simulink model "QC_Test2"  (R2019a)
settings: Solver=FixedStepAuto  StartTime=0.0  StopTime=inf  RelTol=1e-3  EnableMultiTasking=on
libraries: arduinolib x8, simulink x6
settings Model: SimulationMode=external  ExtModeTrigDuration=2  Creator=chait  LastModifiedBy=DINESH
settings OptimizationCC: EnhancedBackFolding=on  PassReuseOutputArgsAs=Individual arguments  MaxStackSize=64  OptimizeBlockOrder=speed  DifferentSizesBufferReuse=on  OptimizationCustomize=off
settings DebuggingCC: ParameterTunabilityLossMsg=error
settings HardwareCC: ProdBitPerInt=16  ProdBitPerPointer=16  ProdBitPerSizeT=16  ProdBitPerPtrDiffT=16  ProdLargestAtomicFloat=None  ProdWordSize=8  ProdHWDeviceType=Atmel->AVR
settings SFSimCC: MATLABDynamicMemAlloc=off
settings RTWCC: SystemTargetFile=ert.tlc  HardwareBoard=Arduino Mega 2560  TLCOptions=-aInlineSetEventsForThisBaseRateFcn=TLC_FALSE -aSuppressMultiTaskScheduler=TLC_FALSE -aRateBasedStepFcn=1  TemplateMakefile=ert_default_tmf  GenerateReport=on  Toolchain=Arduino AVR  BuildConfiguration=Faster Runs  IncludeHyperlinkInReport=on  LaunchReport=on  GenerateTraceInfo=on  GenerateTraceReport=on  GenerateTraceReportSl=on  GenerateTraceReportSf=on  GenerateTraceReportEml=on
settings CodeAppCC: ForceParamTrailComments=on  IgnoreCustomStorageClasses=off  OperatorAnnotations=on  SimulinkDataObjDesc=on  SFDataObjDesc=on  InsertBlockDesc=on
settings ERTTargetCC: SupportContinuousTime=on  SupportVariableSizeSignals=on  ExtMode=on  ExtModeStaticAllocSize=2048  ExtModeMexArgs='127.0.0.1' 0 17725

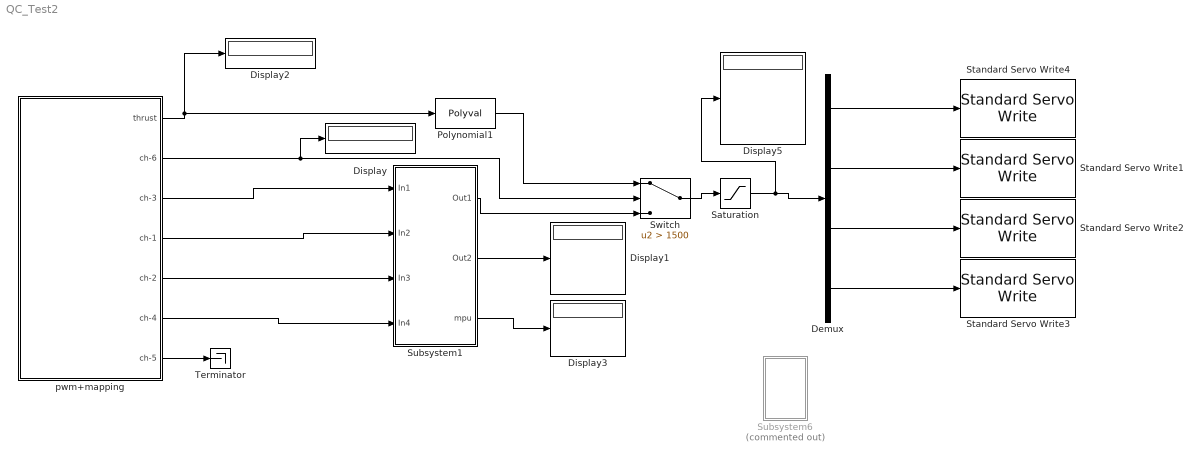
== system QC_Test2 ==
  Demux : Demux
  Display{,1..3,5} (5 alike) : Display
  Polynomial1 : Polyval  Coefs=|
      | [0.097
      |   -52]
  Saturation : Saturate  UpperLimit=142  LowerLimit=45
  Standard Servo Write1 : arduinolib/Standard Servo Write  pinNumber=6  ServoIndex=0  blockPlatform=ARDUINO
      settings: SourceProductName=Simulink Support Package for Arduino Hardware
  Standard Servo Write2 : arduinolib/Standard Servo Write  pinNumber=7  ServoIndex=1  blockPlatform=ARDUINO
      settings: SourceProductName=Simulink Support Package for Arduino Hardware
  Standard Servo Write3 : arduinolib/Standard Servo Write  pinNumber=8  ServoIndex=2  blockPlatform=ARDUINO
      settings: SourceProductName=Simulink Support Package for Arduino Hardware
  Standard Servo Write4 : arduinolib/Standard Servo Write  pinNumber=2  ServoIndex=3  blockPlatform=ARDUINO
      settings: SourceProductName=Simulink Support Package for Arduino Hardware
  Subsystem1 : Subsystem
  Subsystem6 : Subsystem  Commented=on
  Switch : Switch  Criteria=u2 > Threshold  Threshold=1500
  Terminator : Terminator
  pwm+mapping : Subsystem
  wires:
  Subsystem1/1(Out1) -> Switch/3
  Demux/3 -> Standard Servo Write2/1
  Demux/1 -> Standard Servo Write4/1
  pwm+mapping/6(ch-4) -> Subsystem1/4(In4)
  pwm+mapping/5(ch-2) -> Subsystem1/3(In3)
  Subsystem1/3(mpu) -> Display3/1
  pwm+mapping/2(ch-6) -> Display/1, Switch/2
  Polynomial1/1 -> Switch/1
  Switch/1 -> Saturation/1
  Demux/4 -> Standard Servo Write3/1
  Demux/2 -> Standard Servo Write1/1
  Saturation/1 -> Display5/1, Demux/1
  pwm+mapping/3(ch-3) -> Subsystem1/1(In1)
  pwm+mapping/1("thrust ") -> Display2/1, Polynomial1/1
  Subsystem1/2(Out2) -> Display1/1
  pwm+mapping/4(ch-1) -> Subsystem1/2(In2)
  pwm+mapping/7(ch-5) -> Terminator/1

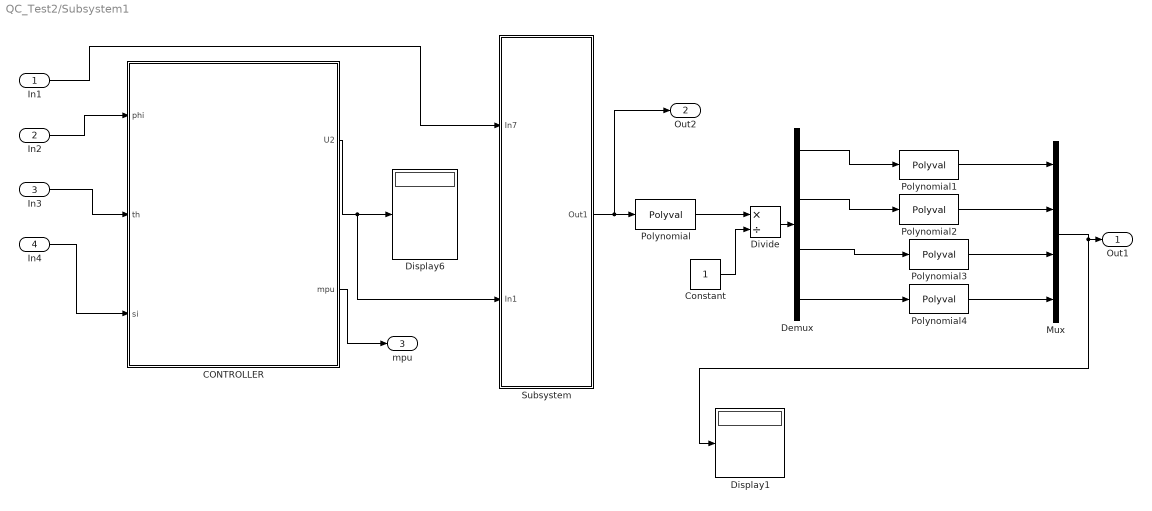
== system QC_Test2/Subsystem1 ==
  In1 : Inport
  In2 : Inport  Port=2
  In3 : Inport  Port=3
  In4 : Inport  Port=4
  CONTROLLER : Subsystem
  Constant : Constant
  Demux : Demux
  Display1 : Display
  Display6 : Display
  Divide : Product  Inputs=*/
  Mux : Mux
  Polynomial : Polyval  Coefs=[1.126e-05 0.05526 1005]
  Polynomial{1..4} (4 alike) : Polyval  Coefs=|
      | [0.097
      |   -52]
  Subsystem : Subsystem
  Out1 : Outport
  Out2 : Outport  Port=2
  mpu : Outport  Port=3
  wires:
  In1/1 -> Subsystem/1(In7)
  Subsystem/1(Out1) -> Out2/1, Polynomial/1
  In2/1 -> CONTROLLER/1(phi)
  In3/1 -> CONTROLLER/2(th)
  CONTROLLER/1(U2) -> Subsystem/2(In1), Display6/1
  Polynomial/1 -> Divide/1
  Divide/1 -> Demux/1
  Constant/1 -> Divide/2
  In4/1 -> CONTROLLER/3(si)
  Mux/1 -> Display1/1, Out1/1
  Polynomial2/1 -> Mux/2
  Polynomial4/1 -> Mux/4
  Polynomial3/1 -> Mux/3
  Polynomial1/1 -> Mux/1
  Demux/1 -> Polynomial1/1
  Demux/2 -> Polynomial2/1
  Demux/3 -> Polynomial3/1
  Demux/4 -> Polynomial4/1
  CONTROLLER/2(mpu) -> mpu/1

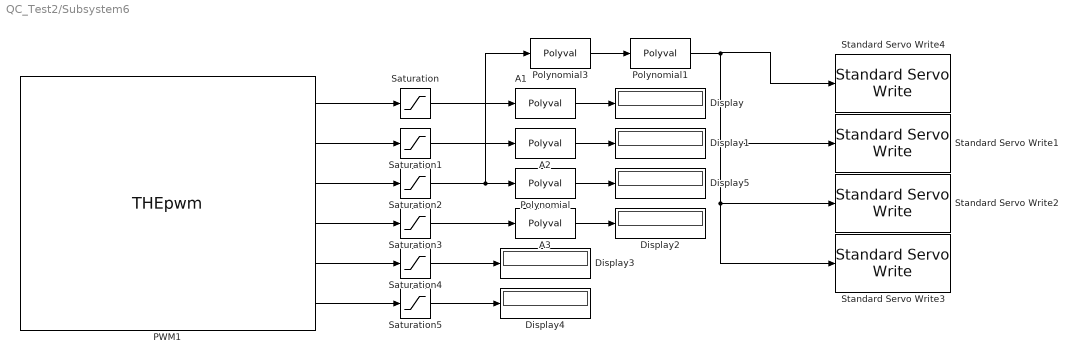
== system QC_Test2/Subsystem6 ==
  A1 : Polyval  Coefs="[0.06  -90]"
  A2 : Polyval  Coefs="[0.06  -90]"
  A3 : Polyval  Coefs="[0.06  -90]"
  Display{,1..5} (6 alike) : Display
  PWM1 : S-Function  InitFcn=try, set_param(gcb,'FunctionName','THEpwm'), end  FunctionName=THEpwm  SFunctionModules=THEpwm_wrapper  SFunctionDeploymentMode=off  EnableBusSupport=off  mask(S-Function Builder){}
      mask help: Simulink:masks:SFunctionBuilder_MD
      mask init:
      | val = [[.9  0.75 0.75 1 1 .9 .9 1]',[1 1 0.75 0.75 .9 .9 1 .9]'];try , sys = get_param(gcb,'SfunBuilderFcnName');if isempty(sys), sys = get_param(gcb,'FunctionName'); end,catch, sys = get_param(gcb,'FunctionName'); end
      settings: CopyFcn=set_param(gcbh,'LinkStatus','none')  PreSaveFcn=try, set_param(gcb,'FunctionName','THEpwm'), end  OpenFcn=sfunctionwizard(gcbh)
      mask Display: plot(val(:,1),val(:,2)),disp(sys), port_label('output',1,'pwm1'), port_label('output',2,'pwm2'), port_label('output',3,'pwm3'), port_label('output',4,'pwm4'), port_label('output',5,'pwm5'), port_label('output',6,'pwm6')
  Polynomial : Polyval  Coefs="[0.02  -20]"
  Polynomial1 : Polyval  Coefs=|
      | [0.097
      |   -52]
  Polynomial3 : Polyval  Coefs=[1.126e-05 0.05526 1005]
  Saturation{,1..5} (6 alike) : Saturate  UpperLimit=2000  LowerLimit=1000
  Standard Servo Write1 : arduinolib/Standard Servo Write  pinNumber=6  ServoIndex=0  blockPlatform=ARDUINO
      settings: SourceProductName=Simulink Support Package for Arduino Hardware
  Standard Servo Write2 : arduinolib/Standard Servo Write  pinNumber=7  ServoIndex=1  blockPlatform=ARDUINO
      settings: SourceProductName=Simulink Support Package for Arduino Hardware
  Standard Servo Write3 : arduinolib/Standard Servo Write  pinNumber=8  ServoIndex=2  blockPlatform=ARDUINO
      settings: SourceProductName=Simulink Support Package for Arduino Hardware
  Standard Servo Write4 : arduinolib/Standard Servo Write  pinNumber=5  ServoIndex=3  blockPlatform=ARDUINO
      settings: SourceProductName=Simulink Support Package for Arduino Hardware
  wires:
  PWM1/1 -> Saturation/1
  PWM1/2 -> Saturation1/1
  PWM1/3 -> Saturation2/1
  PWM1/4 -> Saturation3/1
  PWM1/5 -> Saturation4/1
  PWM1/6 -> Saturation5/1
  Saturation/1 -> A1/1
  Saturation1/1 -> A2/1
  Saturation3/1 -> A3/1
  A1/1 -> Display/1
  A2/1 -> Display1/1
  A3/1 -> Display2/1
  Saturation4/1 -> Display3/1
  Saturation5/1 -> Display4/1
  Saturation2/1 -> Polynomial3/1, Polynomial/1
  Polynomial/1 -> Display5/1
  Polynomial1/1 -> Standard Servo Write4/1, Standard Servo Write3/1, Standard Servo Write2/1, Standard Servo Write1/1
  Polynomial3/1 -> Polynomial1/1

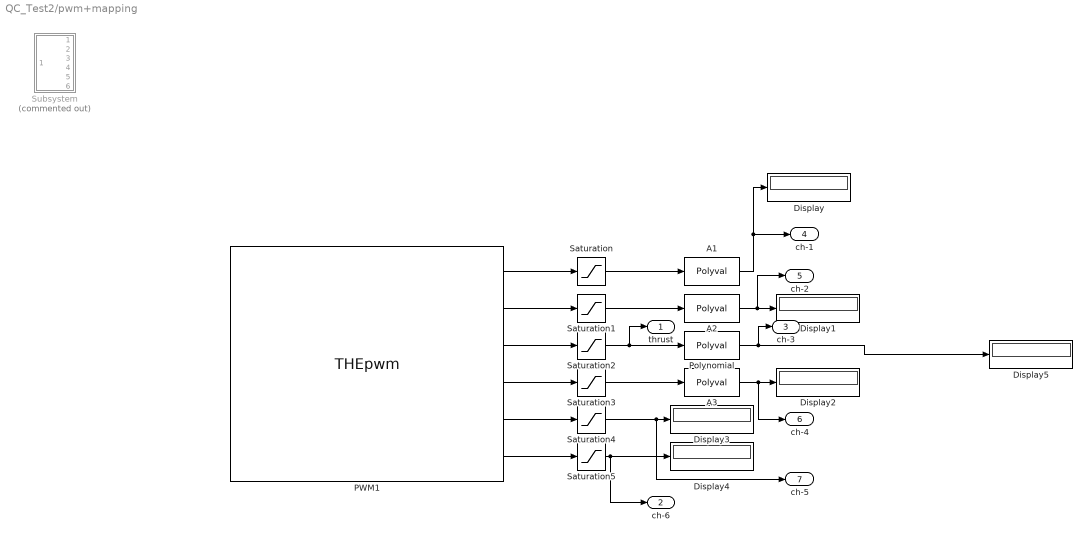
== system QC_Test2/pwm+mapping ==
  A1 : Polyval  Coefs="[0.06  -90]"
  A2 : Polyval  Coefs="[0.06  -90]"
  A3 : Polyval  Coefs="[0.06  -90]"
  Display{,1..5} (6 alike) : Display
  PWM1 : S-Function  InitFcn=try, set_param(gcb,'FunctionName','THEpwm'), end  FunctionName=THEpwm  SFunctionModules=THEpwm_wrapper  SFunctionDeploymentMode=off  EnableBusSupport=off  mask(S-Function Builder){}
      mask help: Simulink:masks:SFunctionBuilder_MD
      mask init: same as QC_Test2/Subsystem6/PWM1
      settings: CopyFcn=set_param(gcbh,'LinkStatus','none')  PreSaveFcn=try, set_param(gcb,'FunctionName','THEpwm'), end  OpenFcn=sfunctionwizard(gcbh)
      mask Display: plot(val(:,1),val(:,2)),disp(sys), port_label('output',1,'pwm1'), port_label('output',2,'pwm2'), port_label('output',3,'pwm3'), port_label('output',4,'pwm4'), port_label('output',5,'pwm5'), port_label('output',6,'pwm6')
  Polynomial : Polyval  Coefs="[0.02  -20]"
  Saturation{,1..5} (6 alike) : Saturate  UpperLimit=2000  LowerLimit=1000
  Subsystem : Subsystem  Commented=on
  "thrust " : Outport
  ch-6 : Outport  Port=2
  ch-3 : Outport  Port=3
  ch-1 : Outport  Port=4
  ch-2 : Outport  Port=5
  ch-4 : Outport  Port=6
  ch-5 : Outport  Port=7
  wires:
  Polynomial/1 -> Display5/1, ch-3/1
  Saturation3/1 -> A3/1
  Saturation/1 -> A1/1
  PWM1/5 -> Saturation4/1
  PWM1/1 -> Saturation/1
  Saturation2/1 -> "thrust "/1, Polynomial/1
  PWM1/4 -> Saturation3/1
  PWM1/6 -> Saturation5/1
  Saturation4/1 -> ch-5/1, Display3/1
  A3/1 -> ch-4/1, Display2/1
  A2/1 -> ch-2/1, Display1/1
  PWM1/3 -> Saturation2/1
  A1/1 -> Display/1, ch-1/1
  PWM1/2 -> Saturation1/1
  Saturation1/1 -> A2/1
  Saturation5/1 -> ch-6/1, Display4/1

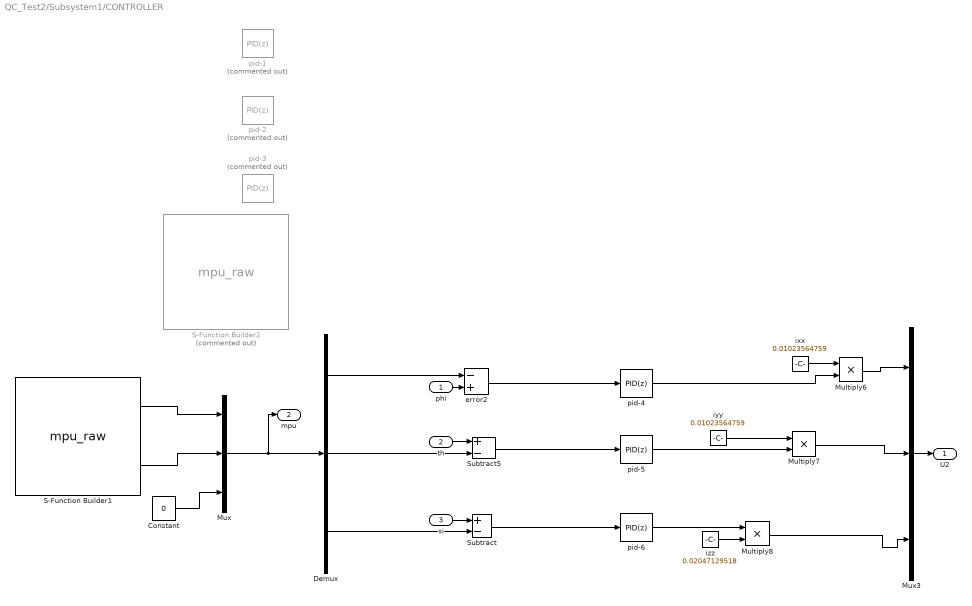
== system QC_Test2/Subsystem1/CONTROLLER ==
  phi : Inport
  th : Inport  Port=2
  si : Inport  Port=3
  Constant : Constant  Value=0
  Demux : Demux  Outputs=3
  Multiply6 : Product  OutDataTypeStr=double
  Multiply7 : Product  OutDataTypeStr=double
  Multiply8 : Product  OutDataTypeStr=double
  Mux : Mux  Inputs=3
  Mux3 : Mux  Inputs=3
  S-Function Builder1 : S-Function  InitFcn=try, set_param(gcb,'FunctionName','mpu_raw'), end  FunctionName=mpu_raw  SFunctionModules=mpu_raw_wrapper  SFunctionDeploymentMode=off  EnableBusSupport=off  mask(S-Function Builder){}
      mask help: Simulink:masks:SFunctionBuilder_MD
      mask init: same as QC_Test2/Subsystem6/PWM1
      settings: CopyFcn=set_param(gcbh,'LinkStatus','none')  PreSaveFcn=try, set_param(gcb,'FunctionName','mpu_raw'), end  OpenFcn=sfunctionwizard(gcbh)
      mask Display: plot(val(:,1),val(:,2)),disp(sys), port_label('output',1,'angle_filter_x'), port_label('output',2,'angle_filter_y')
  S-Function Builder2 : S-Function  Commented=on  InitFcn=try, set_param(gcb,'FunctionName','mpu_raw'), end  FunctionName=mpu_raw  SFunctionModules=mpu_raw_wrapper  SFunctionDeploymentMode=off  EnableBusSupport=off  mask(S-Function Builder){}
      mask help: Simulink:masks:SFunctionBuilder_MD
      mask init: same as QC_Test2/Subsystem6/PWM1
      settings: CopyFcn=set_param(gcbh,'LinkStatus','none')  PreSaveFcn=try, set_param(gcb,'FunctionName','mpu_raw'), end  OpenFcn=sfunctionwizard(gcbh)
      mask Display: plot(val(:,1),val(:,2)),disp(sys), port_label('output',1,'angle_filter_x'), port_label('output',2,'angle_filter_y')
  Subtract : Sum  Inputs=+-
  Subtract5 : Sum  Inputs=+-
  error2 : Sum  Inputs=-+
  ixx : Constant  Value=0.01023564759
  iyy : Constant  Value=0.01023564759
  izz : Constant  Value=0.02047129518
  pid-1 : simulink/Continuous/PID Controller  Commented=on  Controller=PID  Form=Parallel  TimeDomain=Discrete-time  SampleTime=-1  IntegratorMethod=Forward Euler  FilterMethod=Forward Euler  ControllerParametersSource=internal  P=74.6713289213923  I=0.375427323113795  D=2581.8927968404  UseFilter=on  N=1.11198054845437  TunerSelectOption=Transfer Function Based (PID Tuner App)  InitialConditionSource=internal  InitialConditionForIntegrator=0  InitialConditionForFilter=0  DifferentiatorICPrevScaledInput=0  ExternalReset=none  TrackingMode=off  Kt=1  LimitOutput=off  UpperSaturationLimit=inf  LowerSaturationLimit=-inf  LinearizeAsGain=off  AntiWindupMode=none  Kb=1  POutMin=[]  POutMax=[]  IOutMin=[]  IOutMax=[]  DOutMin=[]  DOutMax=[]  NOutMin=[]  NOutMax=[]  SumOutMin=[]  SumOutMax=[]  SaturationOutMin=[]  SaturationOutMax=[]  PParamMin=[]  PParamMax=[]  IParamMin=[]  IParamMax=[]  DParamMin=[]  DParamMax=[]  NParamMin=[]  NParamMax=[]  KbParamMin=[]  KbParamMax=[]  KtParamMin=[]  KtParamMax=[]  KbOutMin=[]  KbOutMax=[]  KtOutMin=[]  KtOutMax=[]  IntegratorOutMin=[]  IntegratorOutMax=[]  FilterOutMin=[]  FilterOutMax=[]  SumI1OutMin=[]  SumI1OutMax=[]  SumI2OutMin=[]  SumI2OutMax=[]  SumI3OutMin=[]  SumI3OutMax=[]  SumI4OutMin=[]  SumI4OutMax=[]  SumDOutMin=[]  SumDOutMax=[]  DifferentiatorOutMin=[]  DifferentiatorOutMax=[]  FilterDiffOutCoefMin=[]  FilterDiffOutCoefMax=[]  ReciprocalOutMin=[]  ReciprocalOutMax=[]  SumDenOutMin=[]  SumDenOutMax=[]  SumNumOutMin=[]  SumNumOutMax=[]  DivideOutMin=[]  DivideOutMax=[]  IntegratorContinuousStateAttributes=''  IntegratorStateMustResolveToSignalObject=off  IntegratorRTWStateStorageClass=Auto  FilterContinuousStateAttributes=''  FilterStateMustResolveToSignalObject=off  FilterRTWStateStorageClass=Auto  ParallelPVariant=InternalParameters  IdealPVariant=Disabled  IVariant=InternalParameters  DVariant=InternalParameters  IntegratorVariant=Discrete  SatVariant=Disabled  AWVariant=Passthrough  PCopyVariant=Disabled  TRVariant=Disabled  FdbkBlocksVariant=Forward  IdealPFdbkVariant=Disabled  SatFdbkVariant=Disabled  DerivativeFilterVariant=ForwardEulerFilter  NVariant=InternalParameters  NCopyVariant=Disabled  FilterICVariant=InternalICsFilter  IntegratorICVariant=InternalICs  ExternalResetVariant=Disabled  TRSumVariant=Passthrough  SumFdbkVariant=Disabled  SumVariant=Sum_PID
  pid-2 : simulink/Continuous/PID Controller  Commented=on  Controller=PID  Form=Parallel  TimeDomain=Discrete-time  SampleTime=-1  IntegratorMethod=Forward Euler  FilterMethod=Forward Euler  ControllerParametersSource=internal  P=74.6713289213923  I=0.375427323113795  D=2581.8927968404  UseFilter=on  N=1.11198054845437  TunerSelectOption=Transfer Function Based (PID Tuner App)  InitialConditionSource=internal  InitialConditionForIntegrator=0  InitialConditionForFilter=0  DifferentiatorICPrevScaledInput=0  ExternalReset=none  TrackingMode=off  Kt=1  LimitOutput=off  UpperSaturationLimit=inf  LowerSaturationLimit=-inf  LinearizeAsGain=off  AntiWindupMode=none  Kb=1  POutMin=[]  POutMax=[]  IOutMin=[]  IOutMax=[]  DOutMin=[]  DOutMax=[]  NOutMin=[]  NOutMax=[]  SumOutMin=[]  SumOutMax=[]  SaturationOutMin=[]  SaturationOutMax=[]  PParamMin=[]  PParamMax=[]  IParamMin=[]  IParamMax=[]  DParamMin=[]  DParamMax=[]  NParamMin=[]  NParamMax=[]  KbParamMin=[]  KbParamMax=[]  KtParamMin=[]  KtParamMax=[]  KbOutMin=[]  KbOutMax=[]  KtOutMin=[]  KtOutMax=[]  IntegratorOutMin=[]  IntegratorOutMax=[]  FilterOutMin=[]  FilterOutMax=[]  SumI1OutMin=[]  SumI1OutMax=[]  SumI2OutMin=[]  SumI2OutMax=[]  SumI3OutMin=[]  SumI3OutMax=[]  SumI4OutMin=[]  SumI4OutMax=[]  SumDOutMin=[]  SumDOutMax=[]  DifferentiatorOutMin=[]  DifferentiatorOutMax=[]  FilterDiffOutCoefMin=[]  FilterDiffOutCoefMax=[]  ReciprocalOutMin=[]  ReciprocalOutMax=[]  SumDenOutMin=[]  SumDenOutMax=[]  SumNumOutMin=[]  SumNumOutMax=[]  DivideOutMin=[]  DivideOutMax=[]  IntegratorContinuousStateAttributes=''  IntegratorStateMustResolveToSignalObject=off  IntegratorRTWStateStorageClass=Auto  FilterContinuousStateAttributes=''  FilterStateMustResolveToSignalObject=off  FilterRTWStateStorageClass=Auto  ParallelPVariant=InternalParameters  IdealPVariant=Disabled  IVariant=InternalParameters  DVariant=InternalParameters  IntegratorVariant=Discrete  SatVariant=Disabled  AWVariant=Passthrough  PCopyVariant=Disabled  TRVariant=Disabled  FdbkBlocksVariant=Forward  IdealPFdbkVariant=Disabled  SatFdbkVariant=Disabled  DerivativeFilterVariant=ForwardEulerFilter  NVariant=InternalParameters  NCopyVariant=Disabled  FilterICVariant=InternalICsFilter  IntegratorICVariant=InternalICs  ExternalResetVariant=Disabled  TRSumVariant=Passthrough  SumFdbkVariant=Disabled  SumVariant=Sum_PID
  pid-3 : simulink/Continuous/PID Controller  Commented=on  Controller=PID  Form=Parallel  TimeDomain=Discrete-time  SampleTime=-1  IntegratorMethod=Forward Euler  FilterMethod=Forward Euler  ControllerParametersSource=internal  P=42.5209542040266  I=0.21378390131326  D=1470.23692975561  UseFilter=on  N=1.11198054845437  TunerSelectOption=Transfer Function Based (PID Tuner App)  InitialConditionSource=internal  InitialConditionForIntegrator=0  InitialConditionForFilter=0  DifferentiatorICPrevScaledInput=0  ExternalReset=none  TrackingMode=off  Kt=1  LimitOutput=off  UpperSaturationLimit=inf  LowerSaturationLimit=-inf  LinearizeAsGain=off  AntiWindupMode=none  Kb=1  POutMin=[]  POutMax=[]  IOutMin=[]  IOutMax=[]  DOutMin=[]  DOutMax=[]  NOutMin=[]  NOutMax=[]  SumOutMin=[]  SumOutMax=[]  SaturationOutMin=[]  SaturationOutMax=[]  PParamMin=[]  PParamMax=[]  IParamMin=[]  IParamMax=[]  DParamMin=[]  DParamMax=[]  NParamMin=[]  NParamMax=[]  KbParamMin=[]  KbParamMax=[]  KtParamMin=[]  KtParamMax=[]  KbOutMin=[]  KbOutMax=[]  KtOutMin=[]  KtOutMax=[]  IntegratorOutMin=[]  IntegratorOutMax=[]  FilterOutMin=[]  FilterOutMax=[]  SumI1OutMin=[]  SumI1OutMax=[]  SumI2OutMin=[]  SumI2OutMax=[]  SumI3OutMin=[]  SumI3OutMax=[]  SumI4OutMin=[]  SumI4OutMax=[]  SumDOutMin=[]  SumDOutMax=[]  DifferentiatorOutMin=[]  DifferentiatorOutMax=[]  FilterDiffOutCoefMin=[]  FilterDiffOutCoefMax=[]  ReciprocalOutMin=[]  ReciprocalOutMax=[]  SumDenOutMin=[]  SumDenOutMax=[]  SumNumOutMin=[]  SumNumOutMax=[]  DivideOutMin=[]  DivideOutMax=[]  IntegratorContinuousStateAttributes=''  IntegratorStateMustResolveToSignalObject=off  IntegratorRTWStateStorageClass=Auto  FilterContinuousStateAttributes=''  FilterStateMustResolveToSignalObject=off  FilterRTWStateStorageClass=Auto  ParallelPVariant=InternalParameters  IdealPVariant=Disabled  IVariant=InternalParameters  DVariant=InternalParameters  IntegratorVariant=Discrete  SatVariant=Disabled  AWVariant=Passthrough  PCopyVariant=Disabled  TRVariant=Disabled  FdbkBlocksVariant=Forward  IdealPFdbkVariant=Disabled  SatFdbkVariant=Disabled  DerivativeFilterVariant=ForwardEulerFilter  NVariant=InternalParameters  NCopyVariant=Disabled  FilterICVariant=InternalICsFilter  IntegratorICVariant=InternalICs  ExternalResetVariant=Disabled  TRSumVariant=Passthrough  SumFdbkVariant=Disabled  SumVariant=Sum_PID
  pid-4 : simulink/Continuous/PID Controller  Controller=PID  Form=Parallel  TimeDomain=Discrete-time  SampleTime=-1  IntegratorMethod=Forward Euler  FilterMethod=Forward Euler  ControllerParametersSource=internal  P=1439.75952951604  I=33.0990500762069  D=11436.5808901528  UseFilter=on  N=4.81287153760732  TunerSelectOption=Transfer Function Based (PID Tuner App)  InitialConditionSource=internal  InitialConditionForIntegrator=0  InitialConditionForFilter=0  DifferentiatorICPrevScaledInput=0  ExternalReset=none  TrackingMode=off  Kt=1  LimitOutput=off  UpperSaturationLimit=inf  LowerSaturationLimit=-inf  LinearizeAsGain=off  AntiWindupMode=none  Kb=1  POutMin=[]  POutMax=[]  IOutMin=[]  IOutMax=[]  DOutMin=[]  DOutMax=[]  NOutMin=[]  NOutMax=[]  SumOutMin=[]  SumOutMax=[]  SaturationOutMin=[]  SaturationOutMax=[]  PParamMin=[]  PParamMax=[]  IParamMin=[]  IParamMax=[]  DParamMin=[]  DParamMax=[]  NParamMin=[]  NParamMax=[]  KbParamMin=[]  KbParamMax=[]  KtParamMin=[]  KtParamMax=[]  KbOutMin=[]  KbOutMax=[]  KtOutMin=[]  KtOutMax=[]  IntegratorOutMin=[]  IntegratorOutMax=[]  FilterOutMin=[]  FilterOutMax=[]  SumI1OutMin=[]  SumI1OutMax=[]  SumI2OutMin=[]  SumI2OutMax=[]  SumI3OutMin=[]  SumI3OutMax=[]  SumI4OutMin=[]  SumI4OutMax=[]  SumDOutMin=[]  SumDOutMax=[]  DifferentiatorOutMin=[]  DifferentiatorOutMax=[]  FilterDiffOutCoefMin=[]  FilterDiffOutCoefMax=[]  ReciprocalOutMin=[]  ReciprocalOutMax=[]  SumDenOutMin=[]  SumDenOutMax=[]  SumNumOutMin=[]  SumNumOutMax=[]  DivideOutMin=[]  DivideOutMax=[]  IntegratorContinuousStateAttributes=''  IntegratorStateMustResolveToSignalObject=off  IntegratorRTWStateStorageClass=Auto  FilterContinuousStateAttributes=''  FilterStateMustResolveToSignalObject=off  FilterRTWStateStorageClass=Auto  ParallelPVariant=InternalParameters  IdealPVariant=Disabled  IVariant=InternalParameters  DVariant=InternalParameters  IntegratorVariant=Discrete  SatVariant=Disabled  AWVariant=Passthrough  PCopyVariant=Disabled  TRVariant=Disabled  FdbkBlocksVariant=Forward  IdealPFdbkVariant=Disabled  SatFdbkVariant=Disabled  DerivativeFilterVariant=ForwardEulerFilter  NVariant=InternalParameters  NCopyVariant=Disabled  FilterICVariant=InternalICsFilter  IntegratorICVariant=InternalICs  ExternalResetVariant=Disabled  TRSumVariant=Passthrough  SumFdbkVariant=Disabled  SumVariant=Sum_PID
  pid-5 : simulink/Continuous/PID Controller  Controller=PID  Form=Parallel  TimeDomain=Discrete-time  SampleTime=-1  IntegratorMethod=Forward Euler  FilterMethod=Forward Euler  ControllerParametersSource=internal  P=1439.7595295244  I=33.099050077218  D=11436.5808902209  UseFilter=on  N=4.81287153760732  TunerSelectOption=Transfer Function Based (PID Tuner App)  InitialConditionSource=internal  InitialConditionForIntegrator=0  InitialConditionForFilter=0  DifferentiatorICPrevScaledInput=0  ExternalReset=none  TrackingMode=off  Kt=1  LimitOutput=off  UpperSaturationLimit=inf  LowerSaturationLimit=-inf  LinearizeAsGain=off  AntiWindupMode=none  Kb=1  POutMin=[]  POutMax=[]  IOutMin=[]  IOutMax=[]  DOutMin=[]  DOutMax=[]  NOutMin=[]  NOutMax=[]  SumOutMin=[]  SumOutMax=[]  SaturationOutMin=[]  SaturationOutMax=[]  PParamMin=[]  PParamMax=[]  IParamMin=[]  IParamMax=[]  DParamMin=[]  DParamMax=[]  NParamMin=[]  NParamMax=[]  KbParamMin=[]  KbParamMax=[]  KtParamMin=[]  KtParamMax=[]  KbOutMin=[]  KbOutMax=[]  KtOutMin=[]  KtOutMax=[]  IntegratorOutMin=[]  IntegratorOutMax=[]  FilterOutMin=[]  FilterOutMax=[]  SumI1OutMin=[]  SumI1OutMax=[]  SumI2OutMin=[]  SumI2OutMax=[]  SumI3OutMin=[]  SumI3OutMax=[]  SumI4OutMin=[]  SumI4OutMax=[]  SumDOutMin=[]  SumDOutMax=[]  DifferentiatorOutMin=[]  DifferentiatorOutMax=[]  FilterDiffOutCoefMin=[]  FilterDiffOutCoefMax=[]  ReciprocalOutMin=[]  ReciprocalOutMax=[]  SumDenOutMin=[]  SumDenOutMax=[]  SumNumOutMin=[]  SumNumOutMax=[]  DivideOutMin=[]  DivideOutMax=[]  IntegratorContinuousStateAttributes=''  IntegratorStateMustResolveToSignalObject=off  IntegratorRTWStateStorageClass=Auto  FilterContinuousStateAttributes=''  FilterStateMustResolveToSignalObject=off  FilterRTWStateStorageClass=Auto  ParallelPVariant=InternalParameters  IdealPVariant=Disabled  IVariant=InternalParameters  DVariant=InternalParameters  IntegratorVariant=Discrete  SatVariant=Disabled  AWVariant=Passthrough  PCopyVariant=Disabled  TRVariant=Disabled  FdbkBlocksVariant=Forward  IdealPFdbkVariant=Disabled  SatFdbkVariant=Disabled  DerivativeFilterVariant=ForwardEulerFilter  NVariant=InternalParameters  NCopyVariant=Disabled  FilterICVariant=InternalICsFilter  IntegratorICVariant=InternalICs  ExternalResetVariant=Disabled  TRSumVariant=Passthrough  SumFdbkVariant=Disabled  SumVariant=Sum_PID
  pid-6 : simulink/Continuous/PID Controller  Controller=PID  Form=Parallel  TimeDomain=Discrete-time  SampleTime=-1  IntegratorMethod=Forward Euler  FilterMethod=Forward Euler  ControllerParametersSource=internal  P=819.858838774975  I=18.8479730147405  D=6512.46387742858  UseFilter=on  N=4.81287153760732  TunerSelectOption=Transfer Function Based (PID Tuner App)  InitialConditionSource=internal  InitialConditionForIntegrator=0  InitialConditionForFilter=0  DifferentiatorICPrevScaledInput=0  ExternalReset=none  TrackingMode=off  Kt=1  LimitOutput=off  UpperSaturationLimit=inf  LowerSaturationLimit=-inf  LinearizeAsGain=off  AntiWindupMode=none  Kb=1  POutMin=[]  POutMax=[]  IOutMin=[]  IOutMax=[]  DOutMin=[]  DOutMax=[]  NOutMin=[]  NOutMax=[]  SumOutMin=[]  SumOutMax=[]  SaturationOutMin=[]  SaturationOutMax=[]  PParamMin=[]  PParamMax=[]  IParamMin=[]  IParamMax=[]  DParamMin=[]  DParamMax=[]  NParamMin=[]  NParamMax=[]  KbParamMin=[]  KbParamMax=[]  KtParamMin=[]  KtParamMax=[]  KbOutMin=[]  KbOutMax=[]  KtOutMin=[]  KtOutMax=[]  IntegratorOutMin=[]  IntegratorOutMax=[]  FilterOutMin=[]  FilterOutMax=[]  SumI1OutMin=[]  SumI1OutMax=[]  SumI2OutMin=[]  SumI2OutMax=[]  SumI3OutMin=[]  SumI3OutMax=[]  SumI4OutMin=[]  SumI4OutMax=[]  SumDOutMin=[]  SumDOutMax=[]  DifferentiatorOutMin=[]  DifferentiatorOutMax=[]  FilterDiffOutCoefMin=[]  FilterDiffOutCoefMax=[]  ReciprocalOutMin=[]  ReciprocalOutMax=[]  SumDenOutMin=[]  SumDenOutMax=[]  SumNumOutMin=[]  SumNumOutMax=[]  DivideOutMin=[]  DivideOutMax=[]  IntegratorContinuousStateAttributes=''  IntegratorStateMustResolveToSignalObject=off  IntegratorRTWStateStorageClass=Auto  FilterContinuousStateAttributes=''  FilterStateMustResolveToSignalObject=off  FilterRTWStateStorageClass=Auto  ParallelPVariant=InternalParameters  IdealPVariant=Disabled  IVariant=InternalParameters  DVariant=InternalParameters  IntegratorVariant=Discrete  SatVariant=Disabled  AWVariant=Passthrough  PCopyVariant=Disabled  TRVariant=Disabled  FdbkBlocksVariant=Forward  IdealPFdbkVariant=Disabled  SatFdbkVariant=Disabled  DerivativeFilterVariant=ForwardEulerFilter  NVariant=InternalParameters  NCopyVariant=Disabled  FilterICVariant=InternalICsFilter  IntegratorICVariant=InternalICs  ExternalResetVariant=Disabled  TRSumVariant=Passthrough  SumFdbkVariant=Disabled  SumVariant=Sum_PID
  U2 : Outport
  mpu : Outport  Port=2
  wires:
  Multiply7/1 -> Mux3/2
  Mux3/1 -> U2/1
  izz/1 -> Multiply8/2
  Multiply6/1 -> Mux3/1
  Multiply8/1 -> Mux3/3
  ixx/1 -> Multiply6/1
  iyy/1 -> Multiply7/1
  Demux/2 -> Subtract5/2
  si/1 -> Subtract/1
  Demux/1 -> error2/1
  phi/1 -> error2/2
  Demux/3 -> Subtract/2
  th/1 -> Subtract5/1
  Mux/1 -> mpu/1, Demux/1
  pid-5/1 -> Multiply7/2
  Subtract5/1 -> pid-5/1
  pid-6/1 -> Multiply8/1
  Subtract/1 -> pid-6/1
  error2/1 -> pid-4/1
  pid-4/1 -> Multiply6/2
  Constant/1 -> Mux/3
  S-Function Builder1/1 -> Mux/1
  S-Function Builder1/2 -> Mux/2

== system QC_Test2/Subsystem1/Subsystem ==
  In7 : Inport
  In1 : Inport  Port=2
  Demux1 : Demux  Outputs=3
  MATLAB Function1 : MATLAB Function  TreatAsAtomicUnit=on
  Mux : Mux
  Saturation : Saturate  UpperLimit=7300  LowerLimit=0
  Subsystem1 : Subsystem
  Out1 : Outport
  wires:
  Demux1/2 -> MATLAB Function1/3(t_t)
  Demux1/1 -> MATLAB Function1/2(t_p)
  Demux1/3 -> MATLAB Function1/4(t_s)
  In7/1 -> MATLAB Function1/1(T)
  MATLAB Function1/1(w1_2) -> Subsystem1/1(w1)
  MATLAB Function1/2(w2_2) -> Subsystem1/2(w2)
  MATLAB Function1/3(w3_2) -> Subsystem1/3(w3)
  MATLAB Function1/4(w4_2) -> Subsystem1/4(w4)
  In1/1 -> Demux1/1
  Subsystem1/4(Out5) -> Mux/4
  Subsystem1/1(Out1) -> Mux/1
  Subsystem1/3(Out3) -> Mux/3
  Subsystem1/2(Out2) -> Mux/2
  Saturation/1 -> Out1/1
  Mux/1 -> Saturation/1

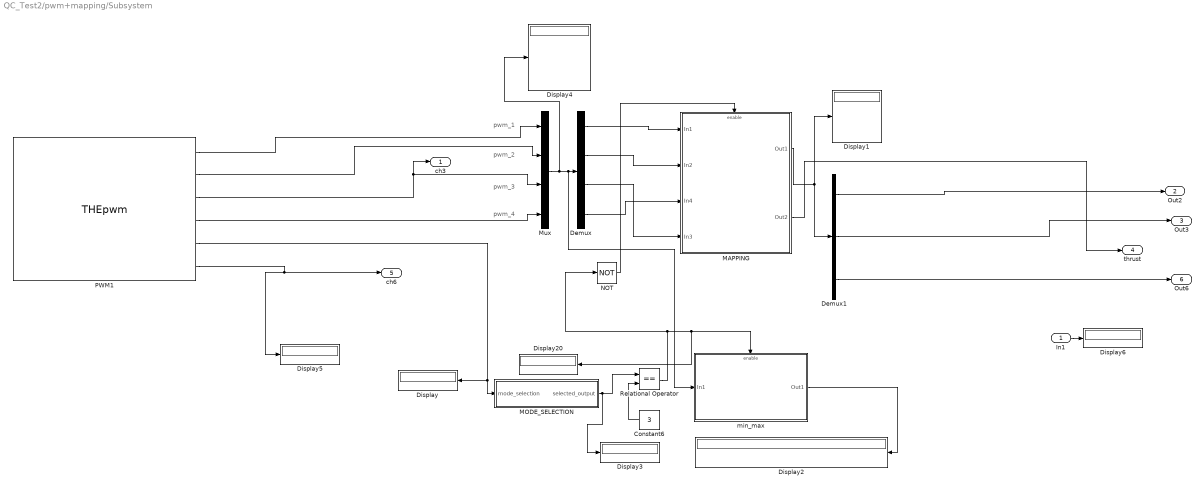
== system QC_Test2/pwm+mapping/Subsystem ==
  note: pwm_2
  note: pwm_3
  note: pwm_4
  note: pwm_1
  In1 : Inport
  Constant6 : Constant  Value=3  OutDataTypeStr=int16
  Demux : Demux
  Demux1 : Demux  Outputs=3
  Display{,1..6,20} (8 alike) : Display
  MAPPING : Subsystem
  MODE_SELECTION : Subsystem
  Mux : Mux
  NOT : Logic  Operator=NOT  IconShape=distinctive  AllPortsSameDT=off  OutDataTypeStr=boolean
  PWM1 : S-Function  InitFcn=try, set_param(gcb,'FunctionName','THEpwm'), end  FunctionName=THEpwm  SFunctionModules=THEpwm_wrapper  SFunctionDeploymentMode=off  EnableBusSupport=off  mask(S-Function Builder){}
      mask help: Simulink:masks:SFunctionBuilder_MD
      mask init: same as QC_Test2/Subsystem6/PWM1
      settings: CopyFcn=set_param(gcbh,'LinkStatus','none')  PreSaveFcn=try, set_param(gcb,'FunctionName','THEpwm'), end  OpenFcn=sfunctionwizard(gcbh)
      mask Display: plot(val(:,1),val(:,2)),disp(sys), port_label('output',1,'pwm1'), port_label('output',2,'pwm2'), port_label('output',3,'pwm3'), port_label('output',4,'pwm4'), port_label('output',5,'pwm5'), port_label('output',6,'pwm6')
  Relational Operator : RelationalOperator  Operator===  OutDataTypeStr=boolean  RndMeth=Simplest
  min_max : Subsystem
  ch3 : Outport
  Out2 : Outport  Port=2
  Out3 : Outport  Port=3
  thrust : Outport  Port=4
  "ch6 " : Outport  Port=5
  Out6 : Outport  Port=6
  wires:
  min_max/1(Out1) -> Display2/1
  Mux/1 -> Display4/1, min_max/1(In1), Demux/1
  Demux1/3 -> Out6/1
  PWM1/3 -> ch3/1, Mux/3
  Demux/3 -> MAPPING/4(In3)
  In1/1 -> Display6/1
  MODE_SELECTION/1(selected_output) -> Display3/1, Relational Operator/1
  PWM1/5 -> MODE_SELECTION/1(mode_selection), Display/1
  MAPPING/1(Out1) -> Demux1/1, Display1/1
  NOT/1 -> MAPPING/Enable
  Demux/2 -> MAPPING/2(In2)
  Constant6/1 -> Relational Operator/2
  Demux/4 -> MAPPING/3(In4)
  Relational Operator/1 -> NOT/1, Display20/1, min_max/Enable
  Demux/1 -> MAPPING/1(In1)
  PWM1/2 -> Mux/2
  MAPPING/2(Out2) -> thrust/1
  PWM1/6 -> "ch6 "/1, Display5/1
  PWM1/1 -> Mux/1
  PWM1/4 -> Mux/4
  Demux1/2 -> Out3/1
  Demux1/1 -> Out2/1

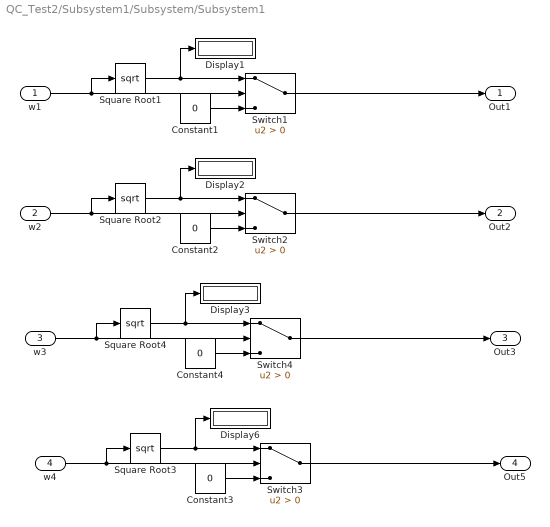
== system QC_Test2/Subsystem1/Subsystem/Subsystem1 ==
  w1 : Inport
  w2 : Inport  Port=2
  w3 : Inport  Port=3
  w4 : Inport  Port=4
  Constant{1..4} (4 alike) : Constant  Value=0
  Display{1..3,6} (4 alike) : Display
  Square Root{1..4} (4 alike) : Sqrt  SaturateOnIntegerOverflow=on
  Switch{1..4} (4 alike) : Switch  Criteria=u2 > Threshold
  Out1 : Outport
  Out2 : Outport  Port=2
  Out3 : Outport  Port=3
  Out5 : Outport  Port=4
  wires:
  Square Root3/1 -> Switch3/1, Display6/1
  Constant3/1 -> Switch3/3
  w4/1 -> Switch3/2, Square Root3/1
  Switch3/1 -> Out5/1
  Square Root1/1 -> Switch1/1, Display1/1
  Switch1/1 -> Out1/1
  Constant1/1 -> Switch1/3
  w1/1 -> Switch1/2, Square Root1/1
  Square Root2/1 -> Switch2/1, Display2/1
  Switch2/1 -> Out2/1
  Constant2/1 -> Switch2/3
  w2/1 -> Switch2/2, Square Root2/1
  Square Root4/1 -> Switch4/1, Display3/1
  Switch4/1 -> Out3/1
  Constant4/1 -> Switch4/3
  w3/1 -> Switch4/2, Square Root4/1

== system QC_Test2/pwm+mapping/Subsystem/MAPPING ==
  In1 : Inport
  In2 : Inport  Port=2
  In4 : Inport  Port=3
  In3 : Inport  Port=4
  Enable : EnablePort
  Subsystem2 : Subsystem
  Out1 : Outport
  Out2 : Outport  Port=2
  wires:
  In1/1 -> Subsystem2/1(roll)
  In3/1 -> Subsystem2/4(yaw)
  Subsystem2/1(Out1) -> Out1/1
  In4/1 -> Subsystem2/3(thrust)
  In2/1 -> Subsystem2/2(pitch)
  Subsystem2/2(Out2) -> Out2/1

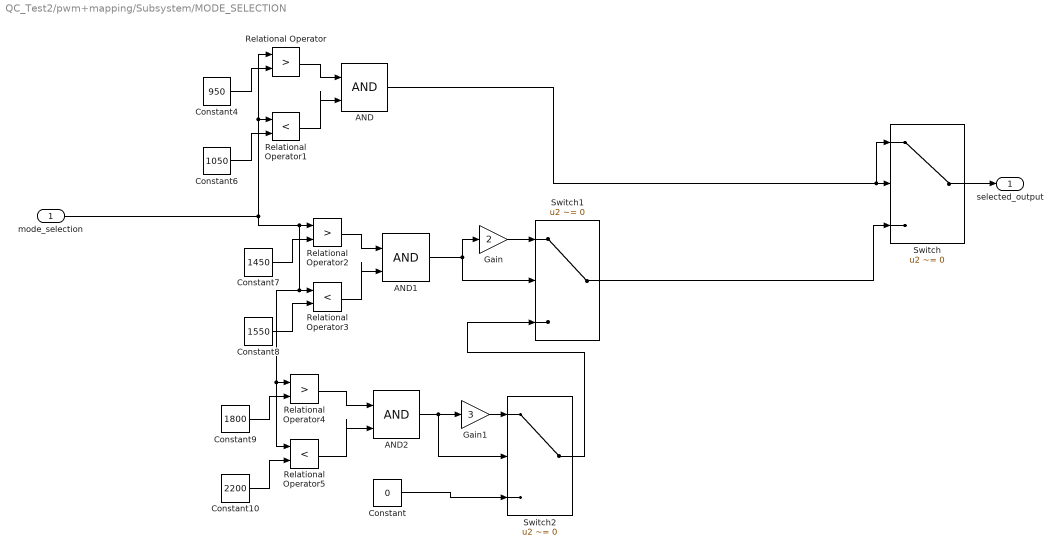
== system QC_Test2/pwm+mapping/Subsystem/MODE_SELECTION ==
  mode_selection : Inport
  AND : Logic  IconShape=distinctive  AllPortsSameDT=off  OutDataTypeStr=boolean
  AND1 : Logic  IconShape=distinctive  AllPortsSameDT=off  OutDataTypeStr=boolean
  AND2 : Logic  IconShape=distinctive  AllPortsSameDT=off  OutDataTypeStr=boolean
  Constant : Constant  Value=0  OutDataTypeStr=single
  Constant10 : Constant  Value=2200  OutDataTypeStr=single
  Constant4 : Constant  Value=950  OutDataTypeStr=single
  Constant6 : Constant  Value=1050  OutDataTypeStr=single
  Constant7 : Constant  Value=1450  OutDataTypeStr=single
  Constant8 : Constant  Value=1550  OutDataTypeStr=single
  Constant9 : Constant  Value=1800  OutDataTypeStr=single
  Gain : Gain  Gain=2
  Gain1 : Gain  Gain=3
  Relational Operator : RelationalOperator  Operator=>  OutDataTypeStr=boolean  RndMeth=Simplest
  Relational Operator1 : RelationalOperator  Operator=<  OutDataTypeStr=boolean  RndMeth=Simplest
  Relational Operator2 : RelationalOperator  Operator=>  OutDataTypeStr=boolean  RndMeth=Simplest
  Relational Operator3 : RelationalOperator  Operator=<  OutDataTypeStr=boolean  RndMeth=Simplest
  Relational Operator4 : RelationalOperator  Operator=>  OutDataTypeStr=boolean  RndMeth=Simplest
  Relational Operator5 : RelationalOperator  Operator=<  OutDataTypeStr=boolean  RndMeth=Simplest
  Switch : Switch  Criteria=u2 ~= 0
  Switch1 : Switch  Criteria=u2 ~= 0
  Switch2 : Switch  Criteria=u2 ~= 0
  selected_output : Outport
  wires:
  mode_selection/1 -> Relational Operator/1, Relational Operator1/1, Relational Operator5/1, Relational Operator4/1, Relational Operator3/1, Relational Operator2/1
  Constant10/1 -> Relational Operator5/2
  Relational Operator4/1 -> AND2/1
  Constant7/1 -> Relational Operator2/2
  Relational Operator5/1 -> AND2/2
  Constant9/1 -> Relational Operator4/2
  Constant8/1 -> Relational Operator3/2
  Relational Operator2/1 -> AND1/1
  Relational Operator3/1 -> AND1/2
  Relational Operator1/1 -> AND/2
  Constant4/1 -> Relational Operator/2
  Relational Operator/1 -> AND/1
  Constant6/1 -> Relational Operator1/2
  AND/1 -> Switch/1, Switch/2
  AND1/1 -> Gain/1, Switch1/2
  AND2/1 -> Switch2/2, Gain1/1
  Switch1/1 -> Switch/3
  Switch2/1 -> Switch1/3
  Constant/1 -> Switch2/3
  Gain/1 -> Switch1/1
  Gain1/1 -> Switch2/1
  Switch/1 -> selected_output/1

== system QC_Test2/pwm+mapping/Subsystem/min_max ==
  In1 : Inport
  Enable : EnablePort
  Subsystem2 : Subsystem
  Out1 : Outport
  wires:
  Subsystem2/1(Output) -> Out1/1
  In1/1 -> Subsystem2/1(In1)

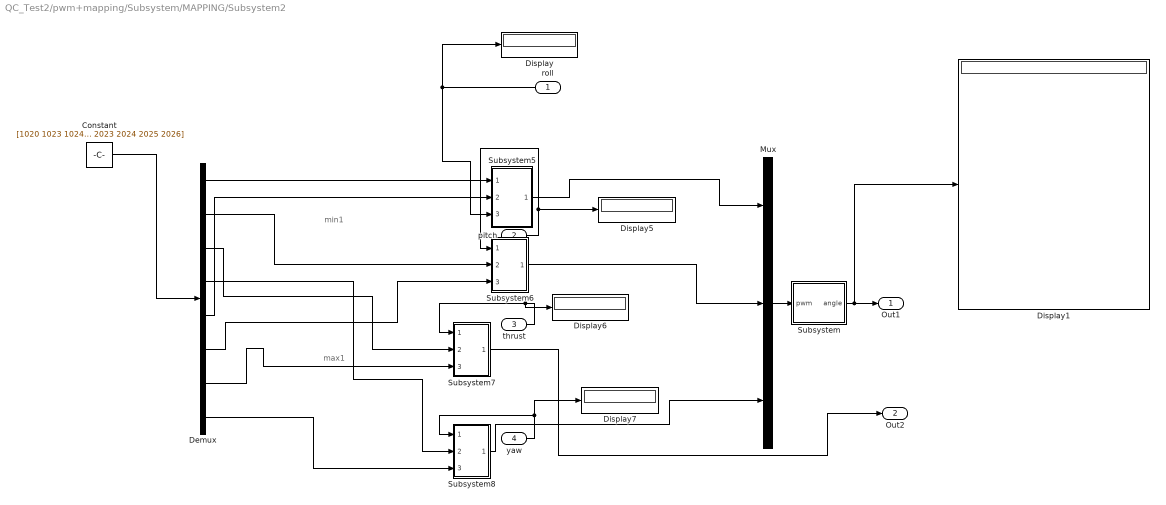
== system QC_Test2/pwm+mapping/Subsystem/MAPPING/Subsystem2 ==
  note: min1
  note: max1
  roll : Inport
  pitch : Inport  Port=2
  thrust : Inport  Port=3
  yaw : Inport  Port=4
  Constant : Constant  Value=[1020 1023 1024 1025 2023 2024 2025 2026]
  Demux : Demux  Outputs=8
  Display{,1,5..7} (5 alike) : Display
  Mux : Mux  Inputs=3
  Subsystem : Subsystem
  Subsystem5 : Subsystem
  Subsystem6 : Subsystem
  Subsystem7 : Subsystem
  Subsystem8 : Subsystem
  Out1 : Outport
  Out2 : Outport  Port=2
  wires:
  roll/1 -> Subsystem5/3("pwm "), Display/1
  Demux/1 -> Subsystem5/1("min ")
  Demux/5 -> Subsystem5/2(max)
  pitch/1 -> Display5/1, Subsystem6/1(pwm_value1)
  Demux/2 -> Subsystem6/2(min)
  Demux/6 -> Subsystem6/3(max)
  thrust/1 -> Subsystem7/1(pwm_value1), Display6/1
  Demux/3 -> Subsystem7/2(min)
  Demux/7 -> Subsystem7/3(max)
  yaw/1 -> Subsystem8/1(pwm_value1), Display7/1
  Demux/4 -> Subsystem8/2(min)
  Demux/8 -> Subsystem8/3(max)
  Subsystem5/1(Out1) -> Mux/1
  Subsystem6/1(Out1) -> Mux/2
  Mux/1 -> Subsystem/1(pwm)
  Subsystem/1(angle) -> Display1/1, Out1/1
  Constant/1 -> Demux/1
  Subsystem8/1(Out1) -> Mux/3
  Subsystem7/1(Out1) -> Out2/1

== system QC_Test2/pwm+mapping/Subsystem/min_max/Subsystem2 ==
  In1 : Inport
  Demux1 : Demux
  Mux2 : Mux  Inputs=8
  S-Function Builder1 : S-Function  InitFcn=try, set_param(gcb,'FunctionName','min_max1'), end  FunctionName=min_max1  SFunctionModules=min_max1_wrapper  SFunctionDeploymentMode=off  EnableBusSupport=off  mask(S-Function Builder){}
      mask help: Simulink:masks:SFunctionBuilder_MD
      mask init: same as QC_Test2/Subsystem6/PWM1
      settings: CopyFcn=set_param(gcbh,'LinkStatus','none')  PreSaveFcn=try, set_param(gcb,'FunctionName','min_max1'), end  OpenFcn=sfunctionwizard(gcbh)
      mask Display:
      | plot(val(:,1),val(:,2))
      | disp(sys)
      | port_label('input',1,'pwm1')
      | port_label('input',2,'pwm2')
      | port_label('input',3,'pwm3')
      | port_label('input',4,'pwm4')
      | port_label('output',1,'min1')
      | port_label('output',2,'min2')
      | port_label('output',3,'min3')
      | port_label('output',4,'min4')
      | port_label('output',5,'max1')
      | port_label('output',6,'max2')
      | port_label('output',7,'max3')
      | port_label('output',8,'max4')
  Output : Outport
  wires:
  Demux1/2 -> S-Function Builder1/2
  S-Function Builder1/5 -> Mux2/5
  Demux1/1 -> S-Function Builder1/1
  S-Function Builder1/7 -> Mux2/7
  Mux2/1 -> Output/1
  S-Function Builder1/1 -> Mux2/1
  S-Function Builder1/6 -> Mux2/6
  Demux1/4 -> S-Function Builder1/4
  S-Function Builder1/3 -> Mux2/3
  Demux1/3 -> S-Function Builder1/3
  S-Function Builder1/4 -> Mux2/4
  S-Function Builder1/8 -> Mux2/8
  In1/1 -> Demux1/1
  S-Function Builder1/2 -> Mux2/2

== system QC_Test2/pwm+mapping/Subsystem/MAPPING/Subsystem2/Subsystem ==
  pwm : Inport
  Add : Sum
  Constant1 : Constant  Value=2000
  Constant2 : Constant  Value=30  OutDataTypeStr=single
  Data Type Conversion1 : DataTypeConversion  OutDataTypeStr=single  SaturateOnIntegerOverflow=on
  Data Type Conversion2 : DataTypeConversion  OutDataTypeStr=single  SaturateOnIntegerOverflow=on
  Data Type Conversion3 : DataTypeConversion  OutDataTypeStr=single  SaturateOnIntegerOverflow=on
  Gain : Gain  Gain=0.06
  Subtract : Sum  Inputs=+-
  angle : Outport
  wires:
  Constant1/1 -> Data Type Conversion2/1
  Gain/1 -> Add/1
  Constant2/1 -> Add/2
  Subtract/1 -> Gain/1
  Add/1 -> Data Type Conversion3/1
  pwm/1 -> Data Type Conversion1/1
  Data Type Conversion1/1 -> Subtract/1
  Data Type Conversion2/1 -> Subtract/2
  Data Type Conversion3/1 -> angle/1

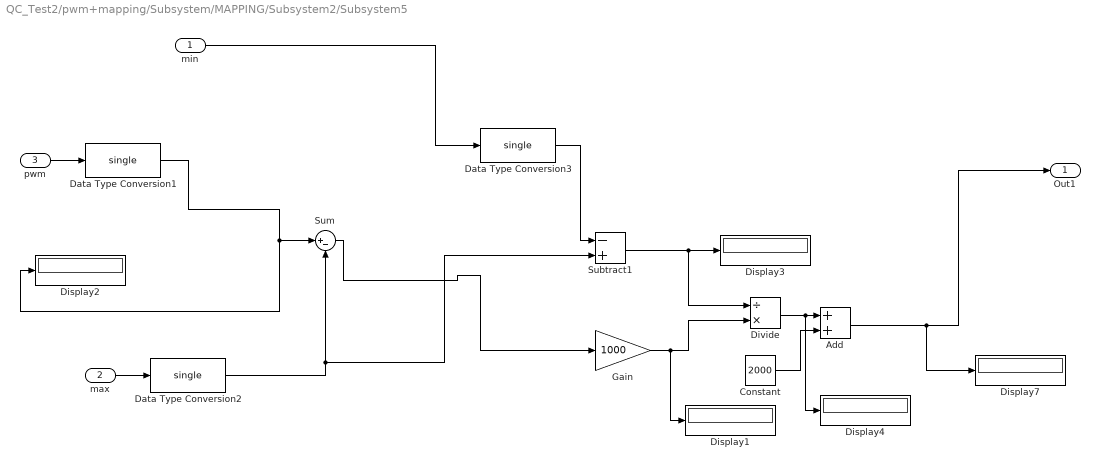
== system QC_Test2/pwm+mapping/Subsystem/MAPPING/Subsystem2/Subsystem5 ==
  "min " : Inport
  max : Inport  Port=2
  "pwm " : Inport  Port=3
  Add : Sum
  Constant : Constant  Value=2000  OutDataTypeStr=single
  Data Type Conversion1 : DataTypeConversion  OutDataTypeStr=single  SaturateOnIntegerOverflow=on
  Data Type Conversion2 : DataTypeConversion  OutDataTypeStr=single  SaturateOnIntegerOverflow=on
  Data Type Conversion3 : DataTypeConversion  OutDataTypeStr=single  SaturateOnIntegerOverflow=on
  Display{1..4,7} (5 alike) : Display
  Divide : Product  Inputs=/*
  Gain : Gain  Gain=1000
  Subtract1 : Sum  Inputs=-+
  Sum : Sum  Inputs=|+-  RndMeth=Nearest
  Out1 : Outport
  wires:
  Sum/1 -> Gain/1
  Data Type Conversion1/1 -> Sum/1, Display2/1
  Data Type Conversion3/1 -> Subtract1/1
  "pwm "/1 -> Data Type Conversion1/1
  Data Type Conversion2/1 -> Sum/2, Subtract1/2
  Divide/1 -> Display4/1, Add/1
  Subtract1/1 -> Display3/1, Divide/1
  Add/1 -> Display7/1, Out1/1
  Gain/1 -> Display1/1, Divide/2
  "min "/1 -> Data Type Conversion3/1
  Constant/1 -> Add/2
  max/1 -> Data Type Conversion2/1

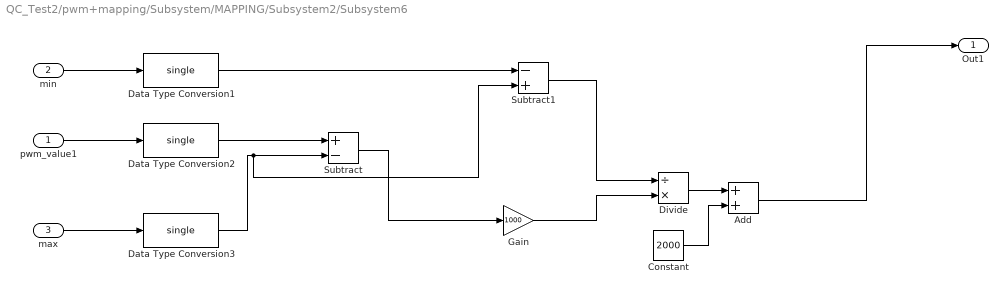
== system QC_Test2/pwm+mapping/Subsystem/MAPPING/Subsystem2/Subsystem6 ==
  pwm_value1 : Inport
  min : Inport  Port=2
  max : Inport  Port=3
  Add : Sum
  Constant : Constant  Value=2000  OutDataTypeStr=single
  Data Type Conversion1 : DataTypeConversion  OutDataTypeStr=single  SaturateOnIntegerOverflow=on
  Data Type Conversion2 : DataTypeConversion  OutDataTypeStr=single  SaturateOnIntegerOverflow=on
  Data Type Conversion3 : DataTypeConversion  OutDataTypeStr=single  SaturateOnIntegerOverflow=on
  Divide : Product  Inputs=/*
  Gain : Gain  Gain=1000
  Subtract : Sum  Inputs=+-
  Subtract1 : Sum  Inputs=-+
  Out1 : Outport
  wires:
  Add/1 -> Out1/1
  pwm_value1/1 -> Data Type Conversion2/1
  max/1 -> Data Type Conversion3/1
  Subtract/1 -> Gain/1
  min/1 -> Data Type Conversion1/1
  Gain/1 -> Divide/2
  Subtract1/1 -> Divide/1
  Divide/1 -> Add/1
  Constant/1 -> Add/2
  Data Type Conversion1/1 -> Subtract1/1
  Data Type Conversion2/1 -> Subtract/1
  Data Type Conversion3/1 -> Subtract1/2, Subtract/2

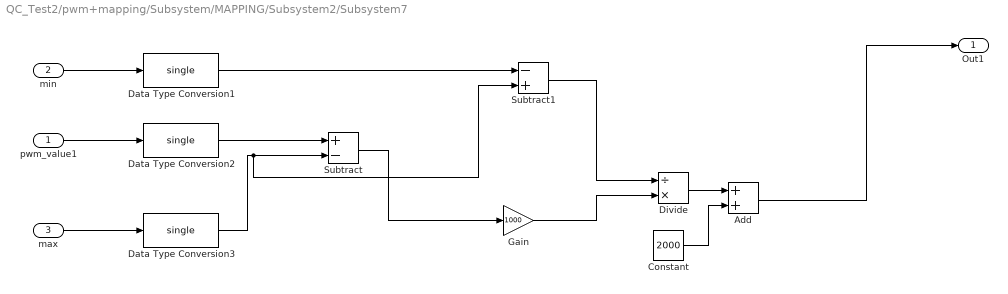
== system QC_Test2/pwm+mapping/Subsystem/MAPPING/Subsystem2/Subsystem7 ==
  pwm_value1 : Inport
  min : Inport  Port=2
  max : Inport  Port=3
  Add : Sum
  Constant : Constant  Value=2000  OutDataTypeStr=single
  Data Type Conversion1 : DataTypeConversion  OutDataTypeStr=single  SaturateOnIntegerOverflow=on
  Data Type Conversion2 : DataTypeConversion  OutDataTypeStr=single  SaturateOnIntegerOverflow=on
  Data Type Conversion3 : DataTypeConversion  OutDataTypeStr=single  SaturateOnIntegerOverflow=on
  Divide : Product  Inputs=/*
  Gain : Gain  Gain=1000
  Subtract : Sum  Inputs=+-
  Subtract1 : Sum  Inputs=-+
  Out1 : Outport
  wires:
  Data Type Conversion1/1 -> Subtract1/1
  Data Type Conversion2/1 -> Subtract/1
  Subtract1/1 -> Divide/1
  max/1 -> Data Type Conversion3/1
  Subtract/1 -> Gain/1
  Divide/1 -> Add/1
  Add/1 -> Out1/1
  pwm_value1/1 -> Data Type Conversion2/1
  min/1 -> Data Type Conversion1/1
  Constant/1 -> Add/2
  Gain/1 -> Divide/2
  Data Type Conversion3/1 -> Subtract1/2, Subtract/2

== system QC_Test2/pwm+mapping/Subsystem/MAPPING/Subsystem2/Subsystem8 ==
  pwm_value1 : Inport
  min : Inport  Port=2
  max : Inport  Port=3
  Add : Sum
  Constant : Constant  Value=2000  OutDataTypeStr=single
  Data Type Conversion1 : DataTypeConversion  OutDataTypeStr=single  SaturateOnIntegerOverflow=on
  Data Type Conversion2 : DataTypeConversion  OutDataTypeStr=single  SaturateOnIntegerOverflow=on
  Data Type Conversion3 : DataTypeConversion  OutDataTypeStr=single  SaturateOnIntegerOverflow=on
  Divide : Product  Inputs=/*
  Gain : Gain  Gain=1000
  Subtract : Sum  Inputs=+-
  Subtract1 : Sum  Inputs=-+
  Out1 : Outport
  wires:
  Data Type Conversion1/1 -> Subtract1/1
  Data Type Conversion2/1 -> Subtract/1
  Subtract1/1 -> Divide/1
  max/1 -> Data Type Conversion3/1
  Subtract/1 -> Gain/1
  Divide/1 -> Add/1
  Add/1 -> Out1/1
  pwm_value1/1 -> Data Type Conversion2/1
  min/1 -> Data Type Conversion1/1
  Constant/1 -> Add/2
  Gain/1 -> Divide/2
  Data Type Conversion3/1 -> Subtract1/2, Subtract/2

== matlab function QC_Test2/Subsystem1/Subsystem/MATLAB Function1 ==
  data: T input; t_p input; t_t input; t_s input; w1_2 output; w2_2 output; w3_2 output; w4_2 output
function [w1_2,w2_2,w3_2,w4_2] = fcn(T,t_p,t_t,t_s)
% ct = 8.586e-08;
% cq = 4.81e-09;
ct = 8.232*10^-8;
cq = 4.832*10^-9;
d  = 0.162635;%meters
 
 co = [ct ct ct ct;
      -d*ct d*ct d*ct -d*ct;
      -d*ct -d*ct d*ct d*ct;
      -cq cq -cq cq];
 i =  (inv(co));
 im = [T;t_p;t_t;t_s] ;
   w = i*im ; 

   w1_2 = w(1,1);
   w2_2 = w(2,1);
   w3_2 = w(3,1);
   w4_2 = w(4,1);
   
     
   
end
